simulink model "problem1"  (R2020b)
settings: Solver=VariableStepAuto  StartTime=0.0  StopTime=10.0  MaxStep=0.01  RelTol=1e-3
PostLoadFcn:
  | M1=100;
  | K1=50;
  | b=50;
  | M2=100;
  | K12=20;
settings Model: OrderedModelArguments=off  Creator=Varun  LastModifiedBy=Varun

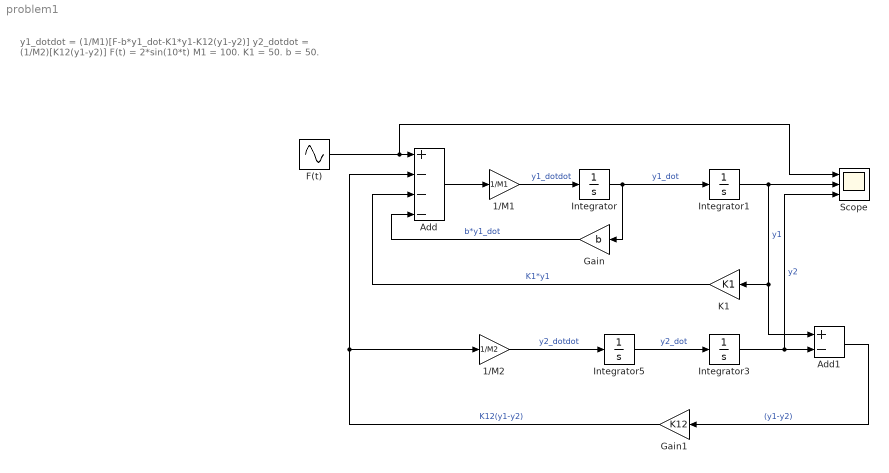
== system problem1 ==
  note: y1_dotdot = (1/M1)[F-b*y1_dot-K1*y1-K12(y1-y2)]
      | y2_dotdot = (1/M2)[K12(y1-y2)]
      | F(t) = 2*sin(10*t)
      | M1 = 100. K1 = 50. b = 50.
  1/M1 : Gain  Gain=1/M1
  1/M2 : Gain  Gain=1/M2
  Add : Sum  Inputs=+---
  Add1 : Sum  Inputs=+-
  F(t) : Sin  Amplitude=2  Frequency=10  SampleTime=0
  Gain : Gain  Gain=b
  Gain1 : Gain  Gain=K12
  Integrator{,1,3,5} (4 alike) : Integrator
  K1 : Gain  Gain=K1
  Scope : Scope  NumInputPorts=3
  wires:
  Integrator/1 -> Gain/1, Integrator1/1  "y1_dot"
  1/M1/1 -> Integrator/1  "y1_dotdot"
  Integrator1/1 -> Scope/2, Add1/1, K1/1  "y1"
  Integrator5/1 -> Integrator3/1  "y2_dot"
  Gain/1 -> Add/4  "b*y1_dot"
  Add/1 -> 1/M1/1
  K1/1 -> Add/3  "K1*y1"
  1/M2/1 -> Integrator5/1  "y2_dotdot"
  Integrator3/1 -> Scope/3, Add1/2  "y2"
  F(t)/1 -> Scope/1, Add/1
  Add1/1 -> Gain1/1  "(y1-y2)"
  Gain1/1 -> 1/M2/1, Add/2  "K12(y1-y2)"
